simulink subsystem "Collect_State_Output"  (R2023a)
settings: Solver=VariableStepAuto  StartTime=0.0  StopTime=10.0  RelTol=1e-3
libraries: nesl_utility x18, sm_lib x1
settings Model: Creator=Andy  LastModifiedBy=Andy

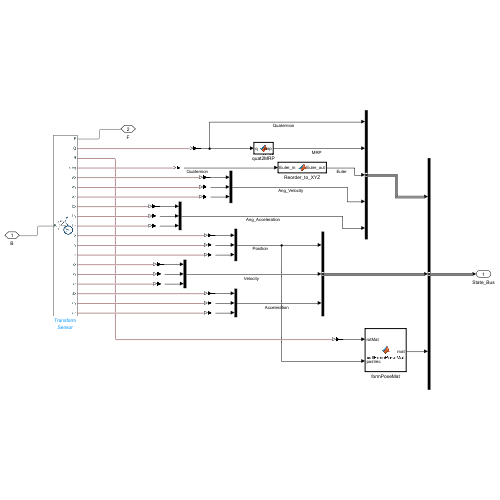
[thumbnail: Simulink's stored preview of the top-level diagram]
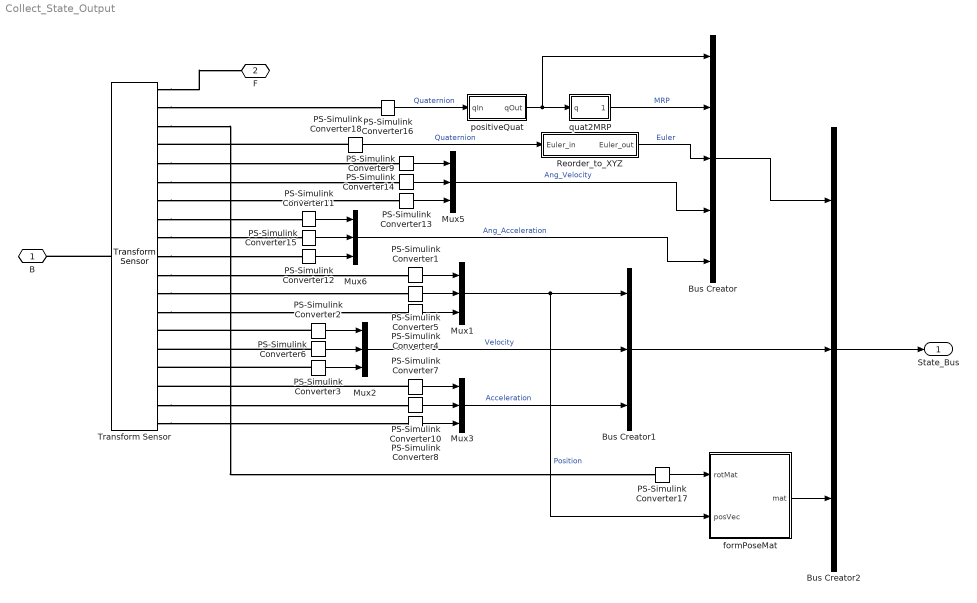
== system Collect_State_Output ==
  Bus Creator : BusCreator  Inputs=5  OutDataTypeStr=Bus: RotStateBus
      settings: InheritFromInputs=off
  Bus Creator1 : BusCreator  Inputs=3  OutDataTypeStr=Bus: TransStateBus
      settings: InheritFromInputs=off
  Bus Creator2 : BusCreator  Inputs=3  OutDataTypeStr=Bus: StateBus
      settings: InheritFromInputs=off
  Mux{1..3,5..6} (5 alike) : Mux  Inputs=3
  PS-Simulink Converter{1..18} (18 alike) : nesl_utility/PS-Simulink Converter  PhysicalDomain=network_engine_domain  SubClassName=ps_output  LeftPortType=input  RightPortType=output  PseudoPeriodic=off  Frequencies=[]  VectorFormat=1-D array  Unit=inherit  AffineConversion=off
  Reorder_to_XYZ : MATLAB Function  TreatAsAtomicUnit=on
  Transform Sensor : sm_lib/Frames and Transforms/Transform Sensor  MeasurementFrame=World  RotationSequence=ZYX  SenseAngle=off  SenseAxis=off  SenseQ=on  SenseR=on  SenseRotationSequence=on  SenseOmegaX=on  SenseOmegaY=on  SenseOmegaZ=on  SenseQDot=off  SenseRDot=off  SenseRotationSequenceDot=off  SenseAlphaX=on  SenseAlphaY=on  SenseAlphaZ=on  SenseQDDot=off  SenseRDDot=off  SenseX=on  SenseY=on  SenseZ=on  SenseRad=off  SenseAzim=off  SenseDist=off  SenseInc=off  SenseXDot=on  SenseYDot=on  SenseZDot=on  SenseRadDot=off  SenseAzimDot=off  SenseDistDot=off  SenseIncDot=off  SenseXDDot=on  SenseYDDot=on  SenseZDDot=on  SenseRadDDot=off  SenseAzimDDot=off  SenseDistDDot=off  SenseIncDDot=off
  formPoseMat : MATLAB Function  TreatAsAtomicUnit=on
  positiveQuat : MATLAB Function  TreatAsAtomicUnit=on
  quat2MRP : MATLAB Function  TreatAsAtomicUnit=on
  B : PMIOPort  Side=Left
  F : PMIOPort  Port=2  Side=Right
  State_Bus : Outport
  wires:
  PS-Simulink Converter4/1 -> Mux1/3
  PS-Simulink Converter5/1 -> Mux1/2
  PS-Simulink Converter1/1 -> Mux1/1
  PS-Simulink Converter3/1 -> Mux2/3
  PS-Simulink Converter6/1 -> Mux2/2
  PS-Simulink Converter2/1 -> Mux2/1
  PS-Simulink Converter10/1 -> Mux3/2
  PS-Simulink Converter8/1 -> Mux3/3
  PS-Simulink Converter7/1 -> Mux3/1
  Mux2/1 -> Bus Creator1/2  "Velocity"
  Mux1/1 -> Bus Creator1/1, formPoseMat/2(posVec)  "Position"
  Mux3/1 -> Bus Creator1/3  "Acceleration"
  PS-Simulink Converter9/1 -> Mux5/1
  PS-Simulink Converter14/1 -> Mux5/2
  PS-Simulink Converter13/1 -> Mux5/3
  Mux5/1 -> Bus Creator/4  "Ang_Velocity"
  PS-Simulink Converter15/1 -> Mux6/2
  PS-Simulink Converter12/1 -> Mux6/3
  Mux6/1 -> Bus Creator/5  "Ang_Acceleration"
  PS-Simulink Converter11/1 -> Mux6/1
  PS-Simulink Converter16/1 -> positiveQuat/1(qIn)  "Quaternion"
  Reorder_to_XYZ/1(Euler_out) -> Bus Creator/3  "Euler"
  Bus Creator/1 -> Bus Creator2/1
  Bus Creator1/1 -> Bus Creator2/2
  Bus Creator2/1 -> State_Bus/1
  PS-Simulink Converter17/1 -> formPoseMat/1(rotMat)
  formPoseMat/1(mat) -> Bus Creator2/3
  quat2MRP/1(mrp) -> Bus Creator/2  "MRP"
  PS-Simulink Converter18/1 -> Reorder_to_XYZ/1(Euler_in)  "Quaternion"
  positiveQuat/1(qOut) -> Bus Creator/1, quat2MRP/1(q)
  connections:
  Transform Sensor/LConn1 -- B/RConn1
  Transform Sensor/RConn1 -- F/RConn1
  Transform Sensor/RConn11 -- PS-Simulink Converter1/LConn1
  Transform Sensor/RConn12 -- PS-Simulink Converter5/LConn1
  Transform Sensor/RConn13 -- PS-Simulink Converter4/LConn1
  PS-Simulink Converter3/LConn1 -- Transform Sensor/RConn16
  PS-Simulink Converter6/LConn1 -- Transform Sensor/RConn15
  PS-Simulink Converter2/LConn1 -- Transform Sensor/RConn14
  Transform Sensor/RConn19 -- PS-Simulink Converter8/LConn1
  PS-Simulink Converter7/LConn1 -- Transform Sensor/RConn17
  Transform Sensor/RConn18 -- PS-Simulink Converter10/LConn1
  Transform Sensor/RConn10 -- PS-Simulink Converter12/LConn1
  Transform Sensor/RConn7 -- PS-Simulink Converter13/LConn1
  Transform Sensor/RConn6 -- PS-Simulink Converter14/LConn1
  Transform Sensor/RConn5 -- PS-Simulink Converter9/LConn1
  Transform Sensor/RConn9 -- PS-Simulink Converter15/LConn1
  Transform Sensor/RConn8 -- PS-Simulink Converter11/LConn1
  Transform Sensor/RConn2 -- PS-Simulink Converter16/LConn1
  Transform Sensor/RConn3 -- PS-Simulink Converter17/LConn1
  PS-Simulink Converter18/LConn1 -- Transform Sensor/RConn4

== matlab function Collect_State_Output/Reorder_to_XYZ ==
  data: Euler_in input; Euler_out output
function Euler_out = reorder_to_xyz(Euler_in)

% Assumes input Euler angles are in yaw-pitch-roll order
% Outputs them in roll-pitch-yaw order
Euler_out = zeros(3,1);
Euler_out(1) = Euler_in(3);
Euler_out(2) = Euler_in(2);
Euler_out(3) = Euler_in(1);

== matlab function Collect_State_Output/formPoseMat ==
  data: rotMat input; mat output; posVec input
function mat  = callFormPoseMat(rotMat,posVec)


[mat] = formPoseMat(rotMat,posVec);

== matlab function Collect_State_Output/positiveQuat ==
  data: qOut output; qIn input
function qOut  = positiveQat(qIn)


if qIn(1) < 0
    qOut = -1.*qIn;
else
    qOut = qIn;
end

== matlab function Collect_State_Output/quat2MRP ==
  data: mrp output; q input
function mrp  = callquatToMRP(q)

[mrp] = quatToMRP(q);
